simulink model "RateModulation"  (R2022a)
settings: Solver=FixedStepAuto  StartTime=0.0  StopTime=inf  FixedStep=1e-3  RelTol=1e-3  EnableMultiTasking=on
undefined symbols (not defined in the file): ATR_CMP_REF_PWM, ATR_GND_CTRL, ATR_PACE_CTRL, D0, D1, D10, D11, D12, D13, D2, D3, D4, D5, D6, D7, D8, D9, FRONTEND_CTRL, Mode, PACE_CHARGE_CTRL, PACE_GND_CTRL, PACING_REF_PWM, PTA0, PTA1, PTA2, PTB23, PTB9, PTC16, PTC17, PTC2, PTC3, PTC4, PTD0, PTD1, PTD2, PTD3, VENT_CMP_REF_PWM, VENT_GND_CTRL, VENT_PACE_CTRL, Z_ATR_CTRL, Z_VENT_CTRL
libraries: frdmk64flib x17, dspstat3 x1
settings Model: SimulationMode=external  ExtModeTrigDuration=5  Creator=22363  LastModifiedBy=Muzam
settings OptimizationCC: EnhancedBackFolding=on  PassReuseOutputArgsAs=Individual arguments  ZeroExternalMemoryAtStartup=off  ZeroInternalMemoryAtStartup=off  MaxStackSize=64  OptimizeBlockOrder=speed  DifferentSizesBufferReuse=on  OptimizationCustomize=off  EfficientTunableParamExpr=on
settings DebuggingCC: ParameterTunabilityLossMsg=error
settings HardwareCC: ProdBitPerPointer=32  ProdBitPerSizeT=32  ProdBitPerPtrDiffT=32  ProdLargestAtomicInteger=Long  ProdLargestAtomicFloat=Double  ProdWordSize=32  ProdHWDeviceType=ARM Compatible->ARM Cortex
settings SFSimCC: MATLABDynamicMemAlloc=off
settings RTWCC: SystemTargetFile=ert.tlc  HardwareBoard=NXP FRDM-K64F  TLCOptions="-aInlineSetEventsForThisBaseRateFcn=TLC_FALSE -aSuppressMultiTaskScheduler=TLC_FALSE  -aRateBasedStepFcn=0"  TemplateMakefile=ert_default_tmf  Toolchain=GNU Tools for ARM Embedded Processors
settings CodeAppCC: ForceParamTrailComments=on  IgnoreCustomStorageClasses=off  OperatorAnnotations=on  SimulinkDataObjDesc=on  SFDataObjDesc=on  InsertBlockDesc=on
settings ERTTargetCC: ExtModeTransport=6  ExtModeMexFile=sendToCommService

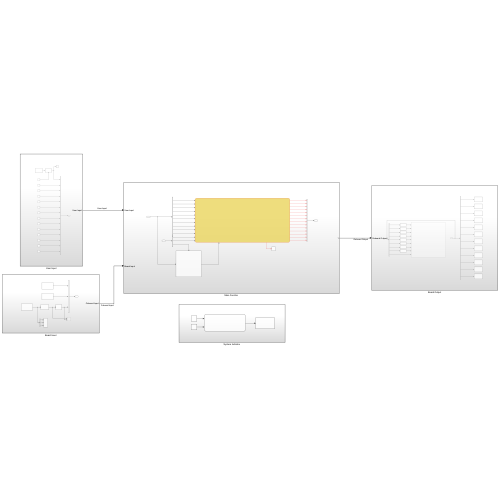
[thumbnail: Simulink's stored preview of the top-level diagram]
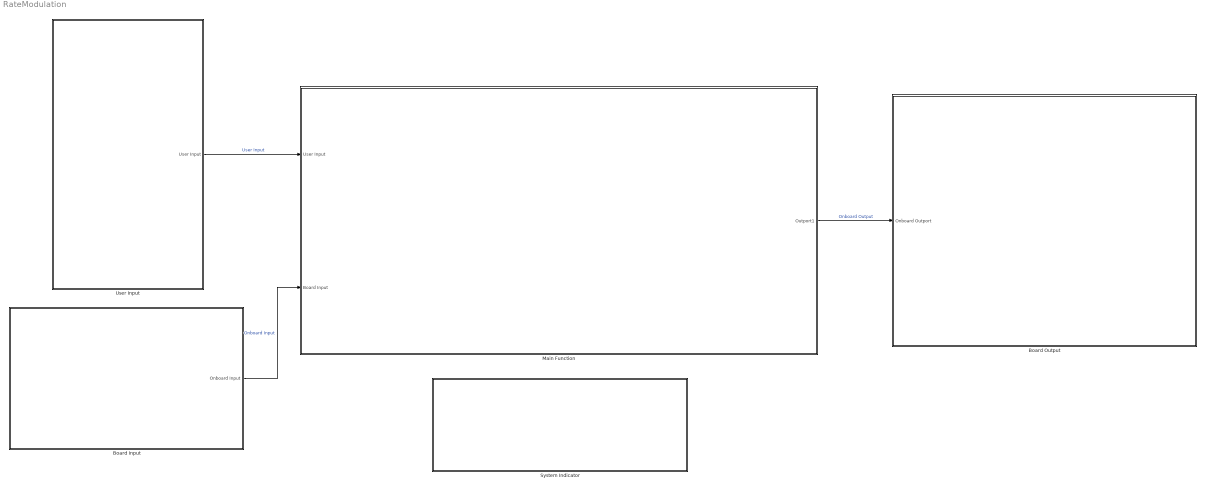
== system RateModulation ==
  Board Input : Subsystem
  Board Output : Subsystem
  Main Function : Subsystem
  System Indicator : Subsystem
  User Input : Subsystem
  wires:
  Main Function/1(Outport1) -> Board Output/1(Onboard Outport)  "Onboard Output"
  User Input/1(User Input) -> Main Function/1(User Input)  "User Input"
  Board Input/1(Onboard Input) -> Main Function/2(Board Input)  "Onboard Input"

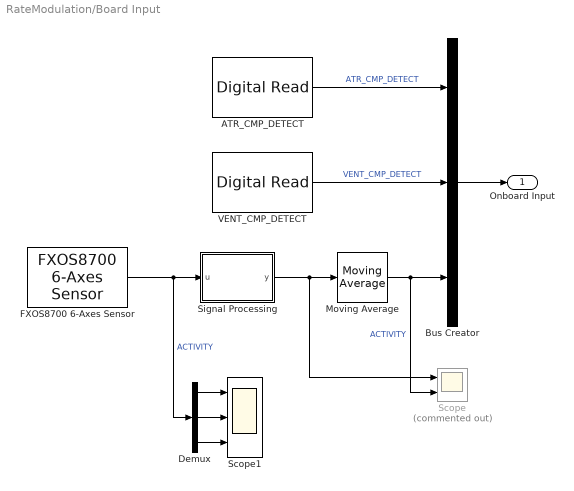
== system RateModulation/Board Input ==
  ATR_CMP_DETECT : frdmk64flib/Digital Read  Whichpin=PTC16 (D0)  SampleTime=-1
  Bus Creator : BusCreator  Inputs=3
  Demux : Demux  Outputs=3
  FXOS8700 6-Axes Sensor : frdmk64flib/FXOS8700 6-Axes Sensor  Activesensor=Accelerometer only  ODR=800Hz  HybridODR=400Hz  Accelfullrange=-4g to +4g  SampleTime=-1
  Moving Average : dspstat3/Moving Average  Method=Sliding window  ForgettingFactorPort=off  SpecifyWindowLength=on  WindowLength=10  ForgettingFactor=0.9  SimulateUsing=Code generation
  Scope : Scope  Commented=on  NumInputPorts=2
  Scope1 : Scope  NumInputPorts=3
  Signal Processing : MATLAB Function  TreatAsAtomicUnit=on
  VENT_CMP_DETECT : frdmk64flib/Digital Read  Whichpin=PTC17 (D1)  SampleTime=-1
  Onboard Input : Outport
  wires:
  VENT_CMP_DETECT/1 -> Bus Creator/2  "VENT_CMP_DETECT"
  ATR_CMP_DETECT/1 -> Bus Creator/1  "ATR_CMP_DETECT"
  Bus Creator/1 -> Onboard Input/1
  FXOS8700 6-Axes Sensor/1 -> Signal Processing/1(u), Demux/1  "ACTIVITY"
  Signal Processing/1(y) -> Moving Average/1, Scope/1
  Demux/1 -> Scope1/1
  Demux/2 -> Scope1/2
  Demux/3 -> Scope1/3
  Moving Average/1 -> Scope/2, Bus Creator/3  "ACTIVITY"

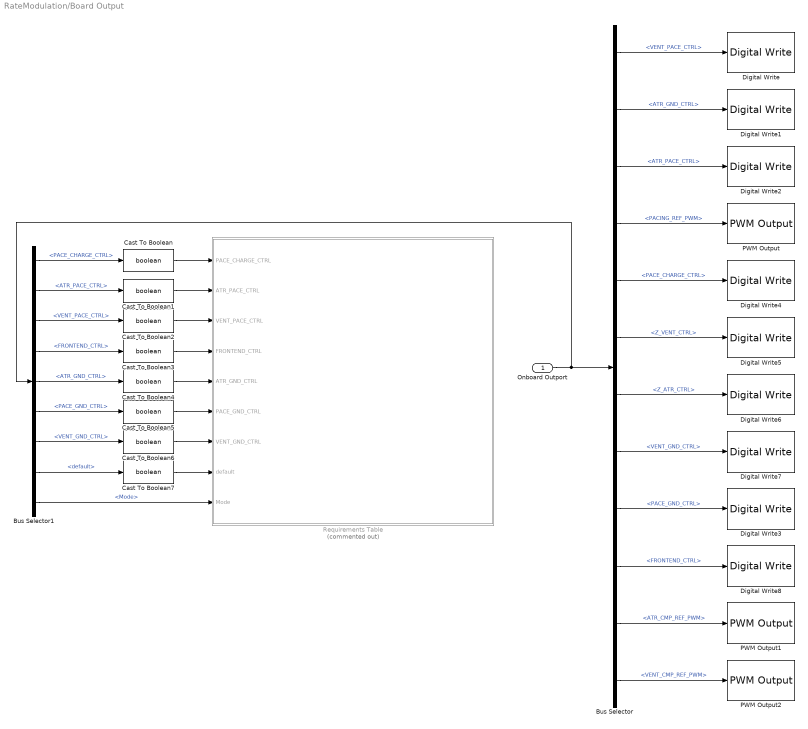
== system RateModulation/Board Output ==
  Onboard Outport : Inport
  Bus Selector : BusSelector  OutputSignals=VENT_PACE_CTRL,ATR_GND_CTRL,ATR_PACE_CTRL,PACING_REF_PWM,PACE_CHARGE_CTRL,Z_VENT_CTRL,Z_ATR_CTRL,VENT_GND_CTRL,PACE_GND_CTRL,FRONTEND_CTRL,ATR_CMP_REF_PWM,VENT_CMP_REF_PWM
  Bus Selector1 : BusSelector  OutputSignals=PACE_CHARGE_CTRL,ATR_PACE_CTRL,VENT_PACE_CTRL,FRONTEND_CTRL,ATR_GND_CTRL,PACE_GND_CTRL,VENT_GND_CTRL,default,Mode
  Cast To Boolean{,1..7} (8 alike) : DataTypeConversion  OutDataTypeStr=boolean  SaturateOnIntegerOverflow=off  RndMeth=Floor
  Digital Write : frdmk64flib/Digital Write  Whichpin=PTC4 (D9)
  Digital Write1 : frdmk64flib/Digital Write  Whichpin=PTD2 (D11)
  Digital Write2 : frdmk64flib/Digital Write  Whichpin=PTA0 (D8)
  Digital Write3 : frdmk64flib/Digital Write  Whichpin=PTD0 (D10)
  Digital Write4 : frdmk64flib/Digital Write  Whichpin=PTB9 (D2)
  Digital Write5 : frdmk64flib/Digital Write  Whichpin=PTC3 (D7)
  Digital Write6 : frdmk64flib/Digital Write  Whichpin=PTB23 (D4)
  Digital Write7 : frdmk64flib/Digital Write  Whichpin=PTD3 (D12)
  Digital Write8 : frdmk64flib/Digital Write  Whichpin=PTD1 (D13)
  PWM Output : frdmk64flib/PWM Output  Whichpin=PTA2 (D5)  InitialFrequency=2000  InitialDutyCycle=50
  PWM Output1 : frdmk64flib/PWM Output  Whichpin=PTC2 (D6)  InitialFrequency=2000  InitialDutyCycle=50
  PWM Output2 : frdmk64flib/PWM Output  Whichpin=PTA1 (D3)  InitialFrequency=2000  InitialDutyCycle=50
  Requirements Table : Requirements Table  Commented=on  TreatAsAtomicUnit=on
  wires:
  Onboard Outport/1 -> Bus Selector1/1, Bus Selector/1
  Bus Selector/1 -> Digital Write/1  "<VENT_PACE_CTRL>"
  Bus Selector/2 -> Digital Write1/1  "<ATR_GND_CTRL>"
  Bus Selector/3 -> Digital Write2/1  "<ATR_PACE_CTRL>"
  Bus Selector/4 -> PWM Output/1  "<PACING_REF_PWM>"
  Bus Selector/5 -> Digital Write4/1  "<PACE_CHARGE_CTRL>"
  Bus Selector/6 -> Digital Write5/1  "<Z_VENT_CTRL>"
  Bus Selector/7 -> Digital Write6/1  "<Z_ATR_CTRL>"
  Bus Selector/8 -> Digital Write7/1  "<VENT_GND_CTRL>"
  Bus Selector/9 -> Digital Write3/1  "<PACE_GND_CTRL>"
  Bus Selector/10 -> Digital Write8/1  "<FRONTEND_CTRL>"
  Bus Selector/11 -> PWM Output1/1  "<ATR_CMP_REF_PWM>"
  Bus Selector/12 -> PWM Output2/1  "<VENT_CMP_REF_PWM>"
  Bus Selector1/9 -> Requirements Table/9(Mode)  "<Mode>"
  Bus Selector1/1 -> Cast To Boolean/1  "<PACE_CHARGE_CTRL>"
  Cast To Boolean/1 -> Requirements Table/1(PACE_CHARGE_CTRL)
  Bus Selector1/2 -> Cast To Boolean1/1  "<ATR_PACE_CTRL>"
  Bus Selector1/3 -> Cast To Boolean2/1  "<VENT_PACE_CTRL>"
  Bus Selector1/4 -> Cast To Boolean3/1  "<FRONTEND_CTRL>"
  Bus Selector1/5 -> Cast To Boolean4/1  "<ATR_GND_CTRL>"
  Bus Selector1/6 -> Cast To Boolean5/1  "<PACE_GND_CTRL>"
  Bus Selector1/7 -> Cast To Boolean6/1  "<VENT_GND_CTRL>"
  Cast To Boolean6/1 -> Requirements Table/7(VENT_GND_CTRL)
  Cast To Boolean5/1 -> Requirements Table/6(PACE_GND_CTRL)
  Cast To Boolean4/1 -> Requirements Table/5(ATR_GND_CTRL)
  Cast To Boolean3/1 -> Requirements Table/4(FRONTEND_CTRL)
  Cast To Boolean2/1 -> Requirements Table/3(VENT_PACE_CTRL)
  Cast To Boolean1/1 -> Requirements Table/2(ATR_PACE_CTRL)
  Bus Selector1/8 -> Cast To Boolean7/1  "<default>"
  Cast To Boolean7/1 -> Requirements Table/8(default)

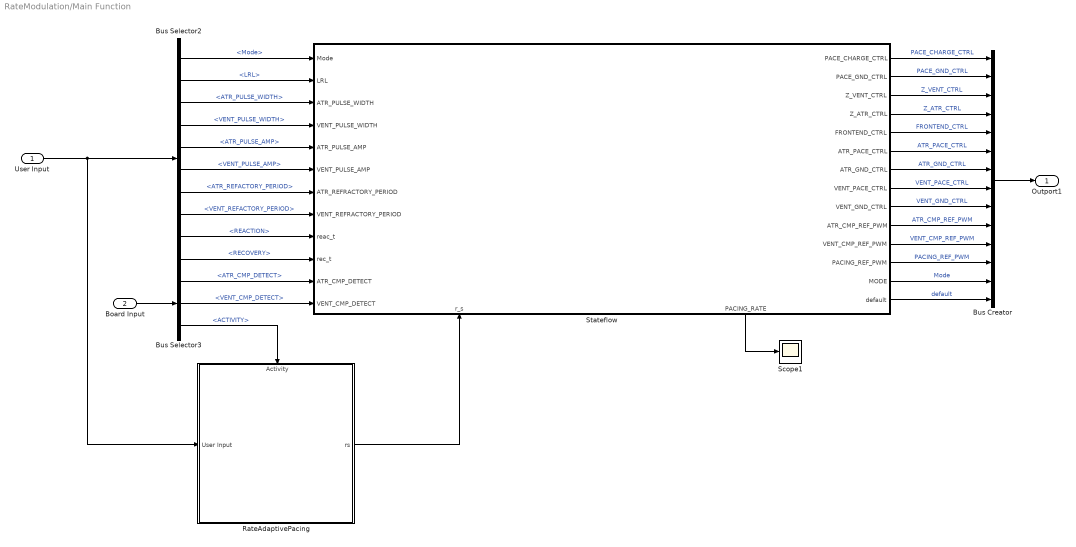
== system RateModulation/Main Function ==
  User Input : Inport
  Board Input : Inport  Port=2
  Bus Creator : BusCreator  Inputs=PACE_CHARGE_CTRL,PACE_GND_CTRL,Z_VENT_CTRL,Z_ATR_CTRL,FRONTEND_CTRL,ATR_PACE_CTRL,ATR_GND_CTRL,VENT_PACE_CTRL,VENT_GND_CTRL,ATR_CMP_REF_PWM,VENT_CMP_REF_PWM,PACING_REF_PWM,Mode,default
  Bus Selector2 : BusSelector  OutputSignals=Mode,LRL,ATR_PULSE_WIDTH,VENT_PULSE_WIDTH,ATR_PULSE_AMP,VENT_PULSE_AMP,ATR_REFACTORY_PERIOD,VENT_REFACTORY_PERIOD,REACTION,RECOVERY
  Bus Selector3 : BusSelector  OutputSignals=ATR_CMP_DETECT,VENT_CMP_DETECT,ACTIVITY
  RateAdaptivePacing : Subsystem
      settings: PortSchema="{\"entries\":[{\"content\":{\"sides\":[{\"content\":{\"connectorIds\":[\"In1\"]},\"type\":\"ConnectorPlacement.EquallySpacedRectSide\",\"uuid\":\"fc785235-65a6-43a6-82c5-cce31898ecd8\"},{\"content\":{\"connectorIds\":[\"Out1\"],\"side\":\"RIGHT\"},\"type\":\"ConnectorPlacement.EquallySpacedRectSide\",\"uuid\":\"d886556e-ae7a-4836-96de-ae0c26c2faa3\"},{\"content\":{\"connectorIds\":[\"In2\"],\"side\":\"TOP\"},\"type\":\"ConnectorPlacement.EquallySpacedRectSide\",\"uuid\":\"9ddfd037-7ca0-48df-974f-64ead127c239\"}]},\"type\":\"ConnectorPlacement.EquallySpacedConnector\",\"uuid\":\"706d4990-08e6-4e14-9b83-9c3b5a55a286\"}],\"packageUris\":[\"http://schema.mathworks.com/mf0/Connector/R2020b\"],\"version\":\"1.0\"}"
  Scope1 : Scope
  Stateflow : Stateflow chart  TreatAsAtomicUnit=on
      settings: PortSchema="{\"entries\":[{\"content\":{\"sides\":[{\"content\":{\"connectorIds\":[\"In1\",\"In2\",\"In3\",\"In4\",\"In5\",\"In6\",\"In7\",\"In8\",\"In9\",\"In10\",\"In11\",\"In12\"]},\"type\":\"ConnectorPlacement.EquallySpacedRectSide\",\"uuid\":\"cedc8d25-7eea-4e97-a354-2884b436d104\"},{\"content\":{\"connectorIds\":[\"Out1\",\"Out2\",\"Out3\",\"Out4\",\"Out5\",\"Out6\",\"Out7\",\"Out8\",\"Out9\",\"Out10\",\"Out11\",\"Out12\",\"Out13\",\"Out14\"],\"side\":\"RIGHT\"},\"type\":\"ConnectorPlacement.EquallySpacedRectSide\",\"uuid\":\"1402aa9e-ac3a-4bcb-a3b3-cabd46d58923\"},{\"content\":{\"connectorIds\":[],\"side\":\"TOP\"},\"type\":\"ConnectorPlacement.EquallySpacedRectSide\",\"uuid\":\"78277392-5036-4a65-906b-e9cf755bf780\"},{\"content\":{\"connectorIds\":[\"In13\",\"Out15\"],\"side\":\"BOTTOM\"},\"type\":\"ConnectorPlacement.EquallySpacedRectSide\",\"uuid\":\"0810e3df-ba89-4942-afb1-d0daac70b0cc\"}]},\"type\":\"ConnectorPlacement.EquallySpacedConnector\",\"uuid\":\"d1c3ca6e-4ee0-4aa3-a542-c9ee957d92b8\"}],\"packageUris\":[\"http://schema.mathworks.com/mf0/Connector/R2020b\"],\"version\":\"1.0\"}"
  Outport1 : Outport
  wires:
  Bus Selector3/2 -> Stateflow/12(VENT_CMP_DETECT)  "<VENT_CMP_DETECT>"
  Bus Selector2/2 -> Stateflow/2(LRL)  "<LRL>"
  Bus Selector2/3 -> Stateflow/3(ATR_PULSE_WIDTH)  "<ATR_PULSE_WIDTH>"
  Bus Selector2/8 -> Stateflow/8(VENT_REFRACTORY_PERIOD)  "<VENT_REFACTORY_PERIOD>"
  Bus Selector2/1 -> Stateflow/1(Mode)  "<Mode>"
  Bus Selector3/1 -> Stateflow/11(ATR_CMP_DETECT)  "<ATR_CMP_DETECT>"
  Bus Selector2/6 -> Stateflow/6(VENT_PULSE_AMP)  "<VENT_PULSE_AMP>"
  Bus Selector2/5 -> Stateflow/5(ATR_PULSE_AMP)  "<ATR_PULSE_AMP>"
  Board Input/1 -> Bus Selector3/1
  User Input/1 -> RateAdaptivePacing/1(User Input), Bus Selector2/1
  Bus Selector2/4 -> Stateflow/4(VENT_PULSE_WIDTH)  "<VENT_PULSE_WIDTH>"
  Bus Selector2/7 -> Stateflow/7(ATR_REFRACTORY_PERIOD)  "<ATR_REFACTORY_PERIOD>"
  Stateflow/1(PACE_CHARGE_CTRL) -> Bus Creator/1  "PACE_CHARGE_CTRL"
  Stateflow/2(PACE_GND_CTRL) -> Bus Creator/2  "PACE_GND_CTRL"
  Stateflow/3(Z_VENT_CTRL) -> Bus Creator/3  "Z_VENT_CTRL"
  Stateflow/4(Z_ATR_CTRL) -> Bus Creator/4  "Z_ATR_CTRL"
  Stateflow/5(FRONTEND_CTRL) -> Bus Creator/5  "FRONTEND_CTRL"
  Stateflow/6(ATR_PACE_CTRL) -> Bus Creator/6  "ATR_PACE_CTRL"
  Stateflow/7(ATR_GND_CTRL) -> Bus Creator/7  "ATR_GND_CTRL"
  Stateflow/8(VENT_PACE_CTRL) -> Bus Creator/8  "VENT_PACE_CTRL"
  Stateflow/9(VENT_GND_CTRL) -> Bus Creator/9  "VENT_GND_CTRL"
  Stateflow/10(ATR_CMP_REF_PWM) -> Bus Creator/10  "ATR_CMP_REF_PWM"
  Stateflow/11(VENT_CMP_REF_PWM) -> Bus Creator/11  "VENT_CMP_REF_PWM"
  Stateflow/12(PACING_REF_PWM) -> Bus Creator/12  "PACING_REF_PWM"
  Stateflow/13(MODE) -> Bus Creator/13  "Mode"
  Stateflow/14(default) -> Bus Creator/14  "default"
  Bus Creator/1 -> Outport1/1
  Bus Selector2/9 -> Stateflow/9(reac_t)  "<REACTION>"
  Bus Selector2/10 -> Stateflow/10(rec_t)  "<RECOVERY>"
  Stateflow/15(PACING_RATE) -> Scope1/1
  Bus Selector3/3 -> RateAdaptivePacing/2(Activity)  "<ACTIVITY>"
  RateAdaptivePacing/1(rs) -> Stateflow/13(r_s)

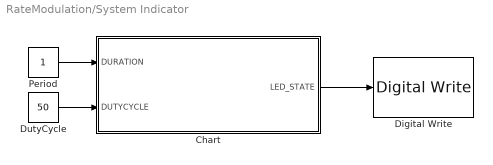
== system RateModulation/System Indicator ==
  Chart : Stateflow chart  TreatAsAtomicUnit=on
  Digital Write : frdmk64flib/Digital Write  Whichpin=RED_LED
  DutyCycle : Constant  Value=50
  Period : Constant
  wires:
  Period/1 -> Chart/1(DURATION)
  Chart/1(LED_STATE) -> Digital Write/1
  DutyCycle/1 -> Chart/2(DUTYCYCLE)

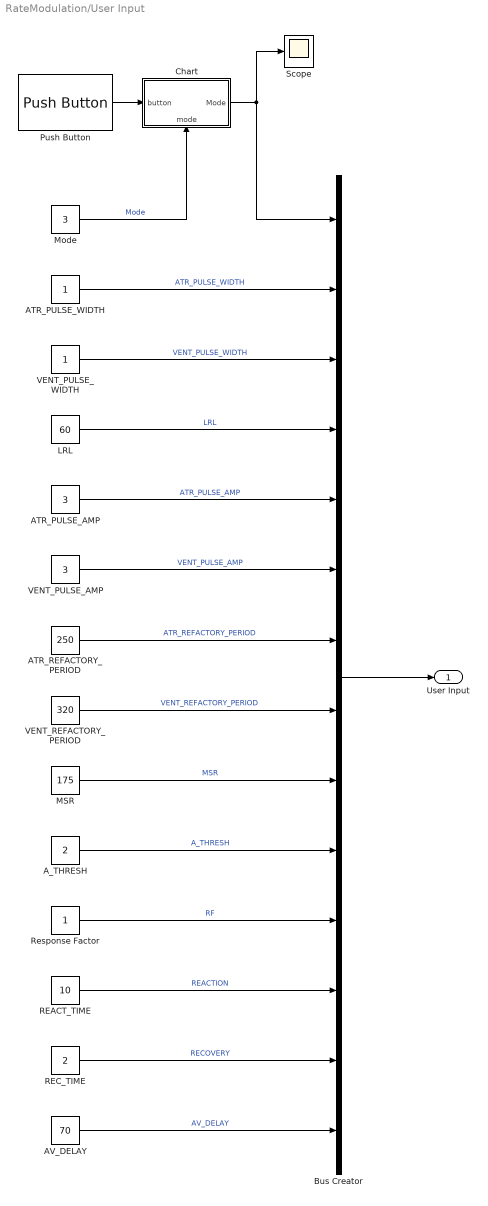
== system RateModulation/User Input ==
  ATR_PULSE_AMP : Constant  Value=3
      settings: AttributesFormatString=0.1-5V
  ATR_PULSE_WIDTH : Constant
      settings: AttributesFormatString=1-30 ms
  ATR_REFACTORY_PERIOD : Constant  Value=250
      settings: AttributesFormatString=150-500 ms
  AV_DELAY : Constant  Value=70
      settings: AttributesFormatString=70-300 ms
  A_THRESH : Constant  Value=2
      settings: AttributesFormatString=|
      | 1 - V_Low   2 - Low   3 - Med_Low
      | 4 - Med   5 - Med_High   6 - High   7 - High
  Bus Creator : BusCreator  Inputs=14
  Chart : Stateflow chart  TreatAsAtomicUnit=on
      settings: PortSchema="{\"entries\":[{\"content\":{\"sides\":[{\"content\":{\"connectorIds\":[\"In2\"]},\"type\":\"ConnectorPlacement.EquallySpacedRectSide\",\"uuid\":\"2e3955a7-e439-432a-a6bd-4b01932f99c2\"},{\"content\":{\"connectorIds\":[\"Out1\"],\"side\":\"RIGHT\"},\"type\":\"ConnectorPlacement.EquallySpacedRectSide\",\"uuid\":\"5e0c39df-00cb-4fe0-963c-53f9b40a1f39\"},{\"content\":{\"connectorIds\":[],\"side\":\"TOP\"},\"type\":\"ConnectorPlacement.EquallySpacedRectSide\",\"uuid\":\"ea7b86d4-657c-4a67-a442-95b269a7616f\"},{\"content\":{\"connectorIds\":[\"In1\"],\"side\":\"BOTTOM\"},\"type\":\"ConnectorPlacement.EquallySpacedRectSide\",\"uuid\":\"3327da06-f30c-459b-ae3c-1030c15cf800\"}]},\"type\":\"ConnectorPlacement.EquallySpacedConnector\",\"uuid\":\"aa69e759-bafe-4cc8-8a1d-6564a6bad6db\"}],\"packageUris\":[\"http://schema.mathworks.com/mf0/Connector/R2020b\"],\"version\":\"1.0\"}"
  LRL : Constant  Value=60
      settings: AttributesFormatString=30-175 ppm
  MSR : Constant  Value=175
      settings: AttributesFormatString=50-175 ppm
  Mode : Constant  Value=3
      settings: AttributesFormatString=|
      | 1 - AOO    3 - AAI    5-8 Rate Modulation
      | 2 - VOO    4 - VVI
  Push Button : frdmk64flib/Push Button  Whichswitch=SW2  SampleTime1=-1
  REACT_TIME : Constant  Value=10
      settings: AttributesFormatString=10-50 s
  REC_TIME : Constant  Value=2
      settings: AttributesFormatString=2-6 min
  Response Factor : Constant
      settings: AttributesFormatString=1-16
  Scope : Scope
  VENT_PULSE_AMP : Constant  Value=3
      settings: AttributesFormatString=0.1-5V
  VENT_PULSE_WIDTH : Constant
      settings: AttributesFormatString=1-30 ms
  VENT_REFACTORY_PERIOD : Constant  Value=320
      settings: AttributesFormatString=150-500 ms
  User Input : Outport
  wires:
  LRL/1 -> Bus Creator/4  "LRL"
  VENT_PULSE_WIDTH/1 -> Bus Creator/3  "VENT_PULSE_WIDTH"
  ATR_PULSE_WIDTH/1 -> Bus Creator/2  "ATR_PULSE_WIDTH"
  Mode/1 -> Chart/1(mode)  "Mode"
  ATR_REFACTORY_PERIOD/1 -> Bus Creator/7  "ATR_REFACTORY_PERIOD"
  VENT_REFACTORY_PERIOD/1 -> Bus Creator/8  "VENT_REFACTORY_PERIOD"
  Bus Creator/1 -> User Input/1
  ATR_PULSE_AMP/1 -> Bus Creator/5  "ATR_PULSE_AMP"
  VENT_PULSE_AMP/1 -> Bus Creator/6  "VENT_PULSE_AMP"
  MSR/1 -> Bus Creator/9  "MSR"
  A_THRESH/1 -> Bus Creator/10  "A_THRESH"
  REACT_TIME/1 -> Bus Creator/12  "REACTION"
  REC_TIME/1 -> Bus Creator/13  "RECOVERY"
  Response Factor/1 -> Bus Creator/11  "RF"
  Push Button/1 -> Chart/2(button)
  Chart/1(Mode) -> Bus Creator/1, Scope/1
  AV_DELAY/1 -> Bus Creator/14  "AV_DELAY"

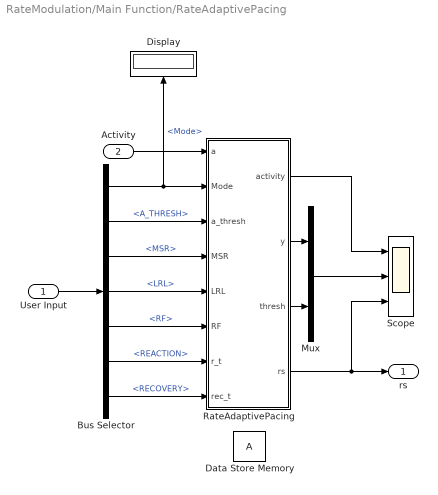
== system RateModulation/Main Function/RateAdaptivePacing ==
  User Input : Inport
  Activity : Inport  Port=2
  Bus Selector : BusSelector  OutputSignals=Mode,A_THRESH,MSR,LRL,RF,REACTION,RECOVERY
  Data Store Memory : DataStoreMemory  WriteAfterWriteMsg=warning  InitialValue=zeros(1,50*800/10)  ShowAdditionalParam=off  OutDataTypeStr=uint8
  Display : Display
  Mux : Mux  Inputs=2
  RateAdaptivePacing : MATLAB Function  TreatAsAtomicUnit=on
  Scope : Scope  NumInputPorts=3
  rs : Outport
  wires:
  Bus Selector/6 -> RateAdaptivePacing/7(r_t)  "<REACTION>"
  Bus Selector/1 -> RateAdaptivePacing/2(Mode), Display/1  "<Mode>"
  RateAdaptivePacing/3(thresh) -> Mux/2
  Bus Selector/2 -> RateAdaptivePacing/3(a_thresh)  "<A_THRESH>"
  RateAdaptivePacing/2(y) -> Mux/1
  Bus Selector/3 -> RateAdaptivePacing/4(MSR)  "<MSR>"
  Bus Selector/7 -> RateAdaptivePacing/8(rec_t)  "<RECOVERY>"
  RateAdaptivePacing/1(activity) -> Scope/1
  Bus Selector/4 -> RateAdaptivePacing/5(LRL)  "<LRL>"
  Bus Selector/5 -> RateAdaptivePacing/6(RF)  "<RF>"
  User Input/1 -> Bus Selector/1
  Mux/1 -> Scope/2
  Activity/1 -> RateAdaptivePacing/1(a)
  RateAdaptivePacing/4(rs) -> rs/1, Scope/3

== stateflow chart RateModulation/Board Output/Requirements Table ==
  (default) -> (junction 1073745504)
  (junction 1073745504) -> (junction 1073745505) : {
      | % SF_REQ_REV_07
      | }
  (junction 1073745505) -> (junction 1073745507) : {
      | % HEADER_ASSIGNMENTS
      |
      | }
  (junction 1073745507) -> (junction 1073745509) : {
      | % START_A_4
      | }
  (junction 1073745509) -> (junction 1073745511) : {
      | }
  (junction 1073745511) -> (junction 1073745513)
  (junction 1073745513) -> (junction 1073745515) : {
      | }
  (junction 1073745515) -> (junction 1073745517) : {
      | % END_A_4
      | }
  (junction 1073745517) -> (junction 1073745519) : {
      | % START_R_22
      | }
  (junction 1073745519) -> (junction 1073745521) : {
      | }
  (junction 1073745521) -> (junction 1073745523)
  (junction 1073745523) -> (junction 1073745525) [order 1] : [(((default) == (1))) && (((FRONTEND_CTRL ) == (0))) && (((PACE_CHARGE_CTRL ) == (0)))]
  (junction 1073745523) -> (junction 1073745531) [order 2]
  (junction 1073745525) -> (junction 1073745527) : {
      | reqtable_postcondition((((PACE_GND_CTRL  ) == (0))) && (((ATR_PACE_CTRL) == (0))) && (((ATR_GND_CTRL ) == (0))) && (((VENT_PACE_CTRL ) == (0))) && (((VENT_GND_CTRL ) == (0))), 'R:1');
      |
      |
      | }
  (junction 1073745527) -> (junction 1073745529) : {
      | }
  (junction 1073745529) -> (junction 1073745531)
  (junction 1073745531) -> (junction 1073745533)
  (junction 1073745533) -> (junction 1073745535) : {
      | % END_R_22
      | }
  (junction 1073745535) -> (junction 1073745537) : {
      | % START_R_1
      | }
  (junction 1073745537) -> (junction 1073745539) : {
      | }
  (junction 1073745539) -> (junction 1073745541)
  (junction 1073745541) -> (junction 1073745543) [order 1] : [(((default) == (0))) && (((Mode) == (1)) || ((Mode) == (3))) && (((PACE_CHARGE_CTRL ) == (0)))]
  (junction 1073745541) -> (junction 1073745549) [order 2]
  (junction 1073745543) -> (junction 1073745545) : {
      | reqtable_postcondition((((PACE_GND_CTRL  ) == (1))) && (((ATR_PACE_CTRL) == (1))) && (((ATR_GND_CTRL ) == (0))) && (((VENT_PACE_CTRL ) == (0))) && (((VENT_GND_CTRL ) == (0))), 'R:2');
      |
      |
      | }
  (junction 1073745545) -> (junction 1073745547) : {
      | }
  (junction 1073745547) -> (junction 1073745549)
  (junction 1073745549) -> (junction 1073745551)
  (junction 1073745551) -> (junction 1073745553) : {
      | % END_R_1
      | }
  (junction 1073745553) -> (junction 1073745555) : {
      | % START_R_7
      | }
  (junction 1073745555) -> (junction 1073745557) : {
      | }
  (junction 1073745557) -> (junction 1073745559)
  (junction 1073745559) -> (junction 1073745561) [order 1] : [(((default) == (0))) && (((Mode) == (2)) || ((Mode) == (4))) && (((PACE_CHARGE_CTRL ) == (0)))]
  (junction 1073745559) -> (junction 1073745567) [order 2]
  (junction 1073745561) -> (junction 1073745563) : {
      | reqtable_postcondition((((PACE_GND_CTRL  ) == (1))) && (((ATR_PACE_CTRL) == (0))) && (((ATR_GND_CTRL ) == (0))) && (((VENT_PACE_CTRL ) == (1))) && (((VENT_GND_CTRL ) == (0))), 'R:3');
      |
      |
      | }
  (junction 1073745563) -> (junction 1073745565) : {
      | }
  (junction 1073745565) -> (junction 1073745567)
  (junction 1073745567) -> (junction 1073745569)
  (junction 1073745569) -> (junction 1073745571) : {
      | % END_R_7
      | }
  (junction 1073745571) -> (junction 1073745573) : {
      | % START_R_25
      | }
  (junction 1073745573) -> (junction 1073745575) : {
      | }
  (junction 1073745575) -> (junction 1073745577)
  (junction 1073745577) -> (junction 1073745579) [order 1] : [(((default) == (0))) && (((Mode) == (1)) || ((Mode) == (3))) && (((FRONTEND_CTRL ) == (1))) && (((PACE_CHARGE_CTRL ) == (1)))]
  (junction 1073745577) -> (junction 1073745585) [order 2]
  (junction 1073745579) -> (junction 1073745581) : {
      | reqtable_postcondition((((PACE_GND_CTRL  ) == (1))) && (((ATR_PACE_CTRL) == (0))) && (((ATR_GND_CTRL ) == (1))) && (((VENT_PACE_CTRL ) == (0))) && (((VENT_GND_CTRL ) == (0))), 'R:4');
      |
      |
      | }
  (junction 1073745581) -> (junction 1073745583) : {
      | }
  (junction 1073745583) -> (junction 1073745585)
  (junction 1073745585) -> (junction 1073745587)
  (junction 1073745587) -> (junction 1073745589) : {
      | % END_R_25
      | }
  (junction 1073745589) -> (junction 1073745591) : {
      | % START_R_28
      | }
  (junction 1073745591) -> (junction 1073745593) : {
      | }
  (junction 1073745593) -> (junction 1073745595)
  (junction 1073745595) -> (junction 1073745597) [order 1] : [(((default) == (0))) && (((Mode) == (2)) || ((Mode) == (4))) && (((FRONTEND_CTRL ) == (1))) && (((PACE_CHARGE_CTRL ) == (1)))]
  (junction 1073745595) -> (junction 1073745603) [order 2]
  (junction 1073745597) -> (junction 1073745599) : {
      | reqtable_postcondition((((PACE_GND_CTRL  ) == (1))) && (((ATR_PACE_CTRL) == (0))) && (((ATR_GND_CTRL ) == (0))) && (((VENT_PACE_CTRL ) == (0))) && (((VENT_GND_CTRL ) == (1))), 'R:5');
      |
      |
      | }
  (junction 1073745599) -> (junction 1073745601) : {
      | }
  (junction 1073745601) -> (junction 1073745603)
  (junction 1073745603) -> (junction 1073745605)
  (junction 1073745605) -> (junction 1073745607) : {
      | % END_R_28
      | }
  (junction 1073745607) -> (junction 1073745609) : {
      | % START_R_31
      | }
  (junction 1073745609) -> (junction 1073745611) : {
      | }
  (junction 1073745611) -> (junction 1073745613)
  (junction 1073745613) -> (junction 1073745615) [order 1] : [(((default) == (0))) && (((Mode) == (1)) || ((Mode) == (3))) && (((PACE_CHARGE_CTRL ) == (1)))]
  (junction 1073745613) -> (junction 1073745621) [order 2]
  (junction 1073745615) -> (junction 1073745617) : {
      | reqtable_postcondition((((PACE_GND_CTRL  ) == (1))) && (((ATR_PACE_CTRL) == (0))) && (((ATR_GND_CTRL ) == (1))) && (((VENT_PACE_CTRL ) == (0))) && (((VENT_GND_CTRL ) == (0))), 'R:6');
      |
      |
      | }
  (junction 1073745617) -> (junction 1073745619) : {
      | }
  (junction 1073745619) -> (junction 1073745621)
  (junction 1073745621) -> (junction 1073745623)
  (junction 1073745623) -> (junction 1073745625) : {
      | % END_R_31
      | }
  (junction 1073745625) -> (junction 1073745627) : {
      | % START_R_34
      | }
  (junction 1073745627) -> (junction 1073745629) : {
      | }
  (junction 1073745629) -> (junction 1073745631)
  (junction 1073745631) -> (junction 1073745633) [order 1] : [(((default) == (0))) && (((Mode) == (2)) || ((Mode) == (4))) && (((PACE_CHARGE_CTRL ) == (1)))]
  (junction 1073745631) -> (junction 1073745639) [order 2]
  (junction 1073745633) -> (junction 1073745635) : {
      | reqtable_postcondition((((PACE_GND_CTRL  ) == (1))) && (((ATR_PACE_CTRL) == (0))) && (((ATR_GND_CTRL ) == (0))) && (((VENT_PACE_CTRL ) == (0))) && (((VENT_GND_CTRL ) == (1))), 'R:7');
      |
      |
      | }
  (junction 1073745635) -> (junction 1073745637) : {
      | }
  (junction 1073745637) -> (junction 1073745639)
  (junction 1073745639) -> (junction 1073745641)
  (junction 1073745641) -> (junction 1073745643) : {
      | % END_R_34
      | }
  data: PACE_CHARGE_CTRL input; ATR_PACE_CTRL input; VENT_PACE_CTRL input; FRONTEND_CTRL input; ATR_GND_CTRL input; PACE_GND_CTRL input; VENT_GND_CTRL input; default input; Mode input

== stateflow chart RateModulation/Main Function/Stateflow ==
  state RATE_MODULATION
    during:
    if Mode>4&&Mode<=8
    if (r_s>PACING_RATE)
    PACING_RATE=PACING_RATE+(r_s-PACING_RATE)/reac_t;
    elseif (r_s<PACING_RATE)
    PACING_RATE=PACING_RATE+(r_s-PACING_RATE)/(60*rec_t);
    else
    PACING_RATE=r_s;
    end
    end
    state AAI_Mode
      entry:
      ATR_CMP_REF_PWM = 80;
      %
      PACING_REF_PWM = ATR_PULSE_AMP*20;
      PACE_GND_CTRL = 1;
      Z_VENT_CTRL = 0;
      Z_ATR_CTRL = 0;
      %
      FRONTEND_CTRL = 1;
      %
      default = 0;
      state Charge
        entry:
        PACE_CHARGE_CTRL = 1;
        ATR_PACE_CTRL = 0;
        ATR_GND_CTRL = 1;
        FRONTEND_CTRL = 1;
      state Pace
        entry:
        PACE_CHARGE_CTRL = 0;
        ATR_PACE_CTRL = 1;
        ATR_GND_CTRL = 0;
        FRONTEND_CTRL = 0;
      RATE_MODULATION.AAI_Mode.Pace -> RATE_MODULATION.AAI_Mode.Charge : after(ATR_PULSE_WIDTH,msec)
      (default) -> RATE_MODULATION.AAI_Mode.Charge
      RATE_MODULATION.AAI_Mode.Charge -> RATE_MODULATION.AAI_Mode.Charge [order 2] : after(ATR_REFRACTORY_PERIOD,msec)[ATR_CMP_DETECT == true]
      RATE_MODULATION.AAI_Mode.Charge -> RATE_MODULATION.AAI_Mode.Pace [order 1] : after(60*1000/PACING_RATE-ATR_REFRACTORY_PERIOD-ATR_PULSE_WIDTH,msec)
    state AOO_Mode
      entry:
      PACING_REF_PWM = ATR_PULSE_AMP*20;
      PACE_GND_CTRL = 1;
      %
      Z_VENT_CTRL = 0;
      Z_ATR_CTRL = 0;
      %
      default = 0;
      state Charge
        entry:
        PACE_CHARGE_CTRL = 1;
        ATR_PACE_CTRL = 0;
        ATR_GND_CTRL = 1;
      state Pace
        entry:
        PACE_CHARGE_CTRL = 0;
        ATR_PACE_CTRL = 1;
        ATR_GND_CTRL = 0;
      (default) -> RATE_MODULATION.AOO_Mode.Charge
      RATE_MODULATION.AOO_Mode.Pace -> RATE_MODULATION.AOO_Mode.Charge : after(ATR_PULSE_WIDTH,msec)
      RATE_MODULATION.AOO_Mode.Charge -> RATE_MODULATION.AOO_Mode.Pace : after(60*1000/PACING_RATE - ATR_PULSE_WIDTH,msec)
    state OFF
      entry:
      PACE_CHARGE_CTRL = 0;
      PACE_GND_CTRL = 0;
      Z_VENT_CTRL = 0;
      Z_ATR_CTRL = 0;
      %
      FRONTEND_CTRL = 0;
      %
      ATR_PACE_CTRL = 0;
      ATR_GND_CTRL = 0;
      VENT_PACE_CTRL = 0;
      VENT_GND_CTRL = 0;
      %
      PACING_RATE = LRL;
      MODE = Mode;
      default = 1
      exit:
      MODE = Mode;
    state VVI_Mode
      entry:
      VENT_CMP_REF_PWM =80;
      %
      PACING_REF_PWM = VENT_PULSE_AMP*20;
      PACE_GND_CTRL = 1;
      Z_VENT_CTRL = 0;
      Z_ATR_CTRL = 0;
      %
      FRONTEND_CTRL = 1;
      %
      default = 0;
      state Charge
        entry:
        PACE_CHARGE_CTRL = 1;
        VENT_PACE_CTRL = 0;
        VENT_GND_CTRL = 1;
        FRONTEND_CTRL = 1;
      state Pace
        entry:
        PACE_CHARGE_CTRL = 0;
        VENT_PACE_CTRL = 1;
        VENT_GND_CTRL = 0;
        FRONTEND_CTRL = 0;
      RATE_MODULATION.VVI_Mode.Pace -> RATE_MODULATION.VVI_Mode.Charge : after(VENT_PULSE_WIDTH,msec)
      (default) -> RATE_MODULATION.VVI_Mode.Charge
      RATE_MODULATION.VVI_Mode.Charge -> RATE_MODULATION.VVI_Mode.Charge [order 2] : after(VENT_REFRACTORY_PERIOD,msec)[VENT_CMP_DETECT == true]
      RATE_MODULATION.VVI_Mode.Charge -> RATE_MODULATION.VVI_Mode.Pace [order 1] : after(60*1000/PACING_RATE-VENT_REFRACTORY_PERIOD-VENT_PULSE_WIDTH,msec)
    state VOO_Mode
      entry:
      PACING_REF_PWM = VENT_PULSE_AMP*20;
      PACE_GND_CTRL = 1;
      %
      Z_VENT_CTRL = 0;
      Z_ATR_CTRL = 0;
      %
      default = 0;
      state Charge
        entry:
        PACE_CHARGE_CTRL = 1;
        VENT_PACE_CTRL = 0;
        VENT_GND_CTRL = 1;
      state Pace
        entry:
        PACE_CHARGE_CTRL = 0;
        VENT_PACE_CTRL = 1;
        VENT_GND_CTRL = 0;
      (default) -> RATE_MODULATION.VOO_Mode.Charge
      RATE_MODULATION.VOO_Mode.Pace -> RATE_MODULATION.VOO_Mode.Charge : after(VENT_PULSE_WIDTH,msec)
      RATE_MODULATION.VOO_Mode.Charge -> RATE_MODULATION.VOO_Mode.Pace : after(60*1000/PACING_RATE - VENT_PULSE_WIDTH,msec)
    (default) -> OFF
    OFF -> AAI_Mode [order 3] : [mod(Mode-1,4)+1 == 3]
    OFF -> AOO_Mode [order 2] : [mod(Mode-1,4)+1 == 1]
    AOO_Mode -> OFF : [mod(Mode-1,4)+1 == 0]
    AAI_Mode -> OFF : [mod(Mode-1,4)+1 == 0]
    VVI_Mode -> OFF : [mod(Mode-1,4)+1 == 0]
    VOO_Mode -> OFF : [mod(Mode-1,4)+1 == 0]
    OFF -> VOO_Mode [order 4] : [mod(Mode-1,4)+1 == 2]
    OFF -> VVI_Mode [order 1] : [mod(Mode-1,4)+1 == 4]
  (default) -> RATE_MODULATION
  data: PACE_CHARGE_CTRL output; PACE_GND_CTRL output; Z_VENT_CTRL output; Z_ATR_CTRL output; FRONTEND_CTRL output; ATR_PACE_CTRL output; ATR_GND_CTRL output; VENT_PACE_CTRL output; VENT_GND_CTRL output; Mode input; LRL input double =1000; ATR_PULSE_WIDTH input double =0.4; VENT_PULSE_WIDTH input double =0.4; ATR_PULSE_AMP input; VENT_PULSE_AMP input; ATR_REFRACTORY_PERIOD input; VENT_REFRACTORY_PERIOD input; reac_t input; rec_t input; ATR_CMP_DETECT input; VENT_CMP_DETECT input; ATR_CMP_REF_PWM output; VENT_CMP_REF_PWM output; PACING_REF_PWM output; MODE output; default output double; r_s input; PACING_RATE output

== matlab function RateModulation/Main Function/RateAdaptivePacing/RateAdaptivePacing ==
  data: activity output; a input; Mode input; a_thresh input; MSR input; LRL input; RF input; r_t input; A data_store_memory; rec_t input; y output; thresh output; rs output
function [activity, y, thresh, rs] = Algorithm(a, Mode, a_thresh, MSR, LRL, RF, r_t, rec_t)
%% Signal Processing
activity = 4*a;

%% Stores past activity to use in operations
global A;
A(1:end-1) = A(2:end);
A(end) = uint8(activity);

%% Rate Response
thresh = 8*a_thresh;
y = double(0);
if (Mode>4 && Mode<8)
    for i = 0:uint16(r_t*800/10)-1
        if ~isnan(A(end-i))
            y = y+double(A(end-i));
        end
    end
    y = double(y/uint16(r_t*800/10));
    rs = double(expRR(y, a_thresh, MSR, LRL, RF));
else
    rs = LRL;
end

%% Exponential Rate Adaptive Curve
function r_s = expRR(x, a_thresh, MSR, LRL, RF)
    a_t = 8*a_thresh;
    r_s = LRL;
    if (x>a_t)
        r_s = double(-exp(-RF*(x-a_t)/(2*(8-a_thresh))+log(MSR-LRL))+MSR);
    end

== stateflow chart RateModulation/System Indicator/Chart ==
  state LED_ON
    entry:
    LED_STATE=true;
  state LED_OFF
    entry:
    LED_STATE=false;
  LED_OFF -> LED_ON : after(DURATION*(1-DUTYCYCLE/100), sec)
  (default) -> LED_ON
  LED_ON -> LED_OFF : after(DURATION*DUTYCYCLE/100, sec)
  data: LED_STATE output; DURATION input; DUTYCYCLE input

== matlab function RateModulation/Board Input/Signal Processing ==
  data: u input; y output
function y = fcn(u)
y = 8*sqrt(u(1)^2+u(2)^2+(1-u(3))^2);

== stateflow chart RateModulation/User Input/Chart ==
  state Button_Down
    en:
    Mode = 0;
    exit:
    Mode = mod(prev,8)+1;
  state Button_Up
    entry:
    prev = Mode;
  (default) -> Button_Up : {Mode=mode}
  Button_Up -> Button_Down : [button]
  Button_Down -> Button_Up : [~button]
  data: mode input; button input; Mode output; prev local
